simulink subsystem "battery_ss"  (R2022b)
settings: Solver=VariableStepAuto  StartTime=0.0  StopTime=10.0  RelTol=1e-3
model mask{obj=obj.Battery}
  mask prompts: obj "slPart Object:"
libraries: fl_lib x13, nesl_utility x3
settings Model: Creator=GeraldoFranciscodeSo  LastModifiedBy=GeraldoFranciscodeSo

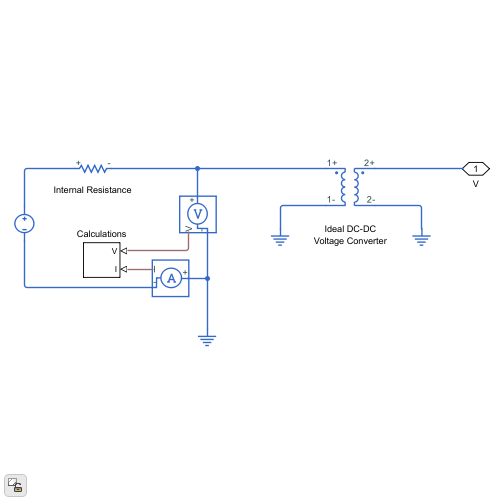
[thumbnail: Simulink's stored preview of the top-level diagram]
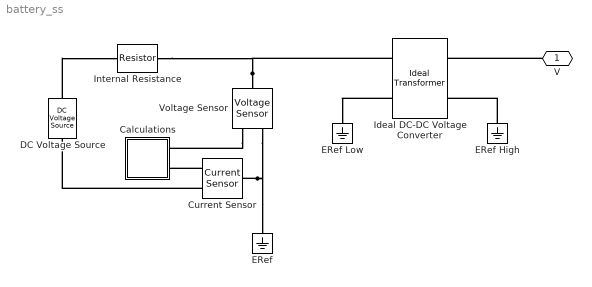
== system battery_ss ==
  Calculations : Subsystem
  Current Sensor : fl_lib/Electrical/Electrical Sensors/Current Sensor
  DC Voltage Source : fl_lib/Electrical/Electrical Sources/DC Voltage Source  v0=obj.BatteryVoltage V
  ERef : fl_lib/Electrical/Electrical Elements/Electrical Reference
  ERef High : fl_lib/Electrical/Electrical Elements/Electrical Reference
  ERef Low : fl_lib/Electrical/Electrical Elements/Electrical Reference
  Ideal DC-DC Voltage Converter : fl_lib/Electrical/Electrical Elements/Ideal Transformer  n=obj.OutputVoltage/obj.BatteryVoltage  i1_specify=off  i1_priority=None  i1=0 A  i1_nominal_specify=off  i1_nominal_unit=A  i1_nominal_value=1  v1_specify=off  v1_priority=None  v1=0 V  v1_nominal_specify=off  v1_nominal_unit=V  v1_nominal_value=1  i2_specify=off  i2_priority=None  i2=0 A  i2_nominal_specify=off  i2_nominal_unit=A  i2_nominal_value=1  v2_specify=off  v2_priority=None  v2=0 V  v2_nominal_specify=off  v2_nominal_unit=V  v2_nominal_value=1
  Internal Resistance : fl_lib/Electrical/Electrical Elements/Resistor  R=0.05 Ohm  i_specify=off  i_priority=High  i=0 A  i_nominal_specify=off  i_nominal_unit=A  i_nominal_value=1  v_specify=off  v_priority=High  v=0 V  v_nominal_specify=off  v_nominal_unit=V  v_nominal_value=1
  Voltage Sensor : fl_lib/Electrical/Electrical Sensors/Voltage Sensor
  V : PMIOPort  Side=Right
  connections:
  Current Sensor/LConn1 -- Voltage Sensor/RConn2 -- ERef/LConn1
  Voltage Sensor/LConn1 -- Ideal DC-DC Voltage Converter/LConn1 -- Internal Resistance/RConn1
  Current Sensor/RConn2 -- DC Voltage Source/RConn1
  Ideal DC-DC Voltage Converter/LConn2 -- ERef Low/LConn1
  Voltage Sensor/RConn1 -- Calculations/LConn1
  DC Voltage Source/LConn1 -- Internal Resistance/LConn1
  ERef High/LConn1 -- Ideal DC-DC Voltage Converter/RConn2
  Current Sensor/RConn1 -- Calculations/LConn2
  V/RConn1 -- Ideal DC-DC Voltage Converter/RConn1

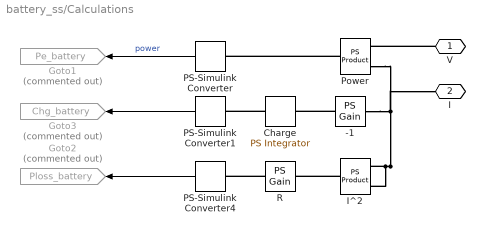
== system battery_ss/Calculations ==
  -1 : fl_lib/Physical Signals/Functions/PS Gain  gain=-1
  Charge : fl_lib/Physical Signals/Linear Operators/PS Integrator  reset_method=foundation.enum.IntegratorResetSpec.None  initial_condition_spec=foundation.enum.IntegratorICSpec.Internal  saturation_spec=foundation.enum.IntegratorSaturationSpec.None  saturation_source_spec=foundation.enum.IntegratorSaturationSourceSpec.Internal  x0=150 A*hr  xu=inf s  xl=-inf s
  Goto1 : Goto  Commented=on  GotoTag=Pe_battery  TagVisibility=global
  Goto2 : Goto  Commented=on  GotoTag=Ploss_battery  TagVisibility=global
  Goto3 : Goto  Commented=on  GotoTag=Chg_battery  TagVisibility=global
  I^2 : fl_lib/Physical Signals/Functions/PS Product
  PS-Simulink Converter : nesl_utility/PS-Simulink Converter  PhysicalDomain=network_engine_domain  SubClassName=ps_output  LeftPortType=input  RightPortType=output  PseudoPeriodic=off  Frequencies=[]  VectorFormat=1-D array  Unit=kW  AffineConversion=off
  PS-Simulink Converter1 : nesl_utility/PS-Simulink Converter  PhysicalDomain=network_engine_domain  SubClassName=ps_output  LeftPortType=input  RightPortType=output  PseudoPeriodic=off  Frequencies=[]  VectorFormat=1-D array  Unit=A*hr  AffineConversion=off
  PS-Simulink Converter4 : nesl_utility/PS-Simulink Converter  PhysicalDomain=network_engine_domain  SubClassName=ps_output  LeftPortType=input  RightPortType=output  PseudoPeriodic=off  Frequencies=[]  VectorFormat=1-D array  Unit=kW  AffineConversion=off
  Power : fl_lib/Physical Signals/Functions/PS Product
  R : fl_lib/Physical Signals/Functions/PS Gain  gain=0.05 V/A
  V : PMIOPort  Side=Left
  I : PMIOPort  Port=2  Side=Left
  wires:
  PS-Simulink Converter/1 -> Goto1/1  "power"
  PS-Simulink Converter1/1 -> Goto3/1
  PS-Simulink Converter4/1 -> Goto2/1
  connections:
  Charge/RConn1 -- PS-Simulink Converter1/LConn1
  Power/RConn1 -- PS-Simulink Converter/LConn1
  V/RConn1 -- Power/LConn1
  I^2/LConn1 -- -1/LConn1 -- Power/LConn2 -- I/RConn1 -- I^2/LConn2
  I^2/RConn1 -- R/LConn1
  R/RConn1 -- PS-Simulink Converter4/LConn1
  -1/RConn1 -- Charge/LConn1
